simulink model "Spange_Thrust_simulation_4mode"  (R2016a)
settings: Solver=ode3  StartTime=0.0  StopTime=4  RelTol=1e-3
values from neighbouring files (symbols this model uses):
  C = [C1;C2;C3]    [Spange_init.m]
  D = 3.0/100    (= 0.03)    [Spange_init.m]
  eps_c = 5    [Spange_init.m]
  epsilon = 0.5    [Spange_init.m]
  hd = c2d(H1,0.1,'foh')    [Spange_init.m]
  hd2 = c2d(H2,0.01,'zoh')    [Spange_init.m]
  I_s = 0.05    [Spange_init.m]
  k_cc = 1    [Spange_init.m]
  K_omega = 0.3    [Spange_init.m]
  K_q1f = 0.0113    [Spange_init.m]
  K_q1r = K_q1f    (= 0.0113)    [Spange_init.m]
  K_q2f = 0.0117    [Spange_init.m]
  K_q2r = K_q2f    (= 0.0117)    [Spange_init.m]
  K_q3f = 0.0113    [Spange_init.m]
  K_q3r = K_q3f    (= 0.0113)    [Spange_init.m]
  K_T1f = 0.3763    [Spange_init.m]
  K_T1r = K_T1f    (= 0.3763)    [Spange_init.m]
  K_T2f = 0.3901    [Spange_init.m]
  K_T2r = K_T2f    (= 0.3901)    [Spange_init.m]
  K_T3f = 0.3776    [Spange_init.m]
  K_T3r = K_T3f    (= 0.3776)    [Spange_init.m]
  Kp = 0.3    [Spange_init.m]
  Max_Acceleration = 2    [Spange_init.m]
  Max_rotation = 12*sqrt(lambda)    [Spange_init.m]
  Max_thrust = 1.5034    [Spange_init.m]
  Min_thrust = -0.85    [Spange_init.m]
  mode = 4    [Spange_init.m]
  n_c = 5    [Spange_init.m]
  n_max = 64.6    [Spange_init.m]
  p_cc = 0.5    [Spange_init.m]
  Q_f0 = 0.3    [Spange_init.m]
  r_cc = 4    [Spange_init.m]
  Rho = Rho_m    (= 1000)    [Spange_init.m]
  td = [1;0;0]    [Spange_init.m]
  Thruster_control = 1    [Spange_init.m]
  ThrusterPosX = [Thruster.T1(1) Thruster.T2(1) Thruster.T3(1)]    [Spange_init.m]
  ThrusterPosY = [Thruster.T1(2) Thruster.T2(2) Thruster.T3(2)]    [Spange_init.m]
  u_e = [1 0 1 0 0 ... (first row only)    [Spange_init.m]
undefined symbols (not defined in the file or in its folder): Thruster
libraries: simulink_extras x16, simulink x8
(part 1 of 3)
settings Model: Creator=Joachim  LastModifiedBy=Joachim
settings DataIOCC: LimitDataPoints=on

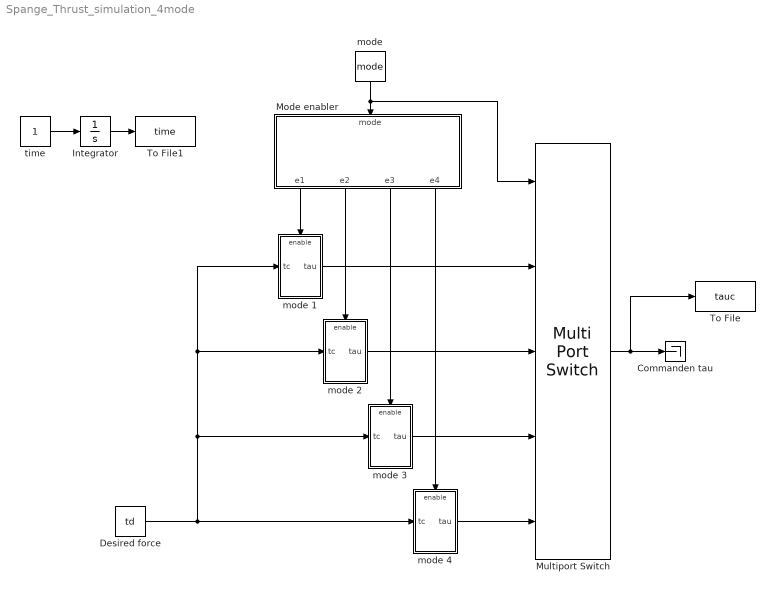
== system Spange_Thrust_simulation_4mode ==
  Commanden tau : Terminator
  Desired force : Constant  Value=td
  Integrator : Integrator
  Mode enabler : MATLAB Function  TreatAsAtomicUnit=on
  Multiport Switch : MultiPortSwitch  Inputs=4
  To File : ToFile  Filename=tauc  SaveFormat=Timeseries
  To File1 : ToFile  Filename=time  SaveFormat=Timeseries
  mode : Constant  Value=mode
  mode 1 : Subsystem
  mode 2 : Subsystem
  mode 3 : Subsystem
  mode 4 : Subsystem
  time : Constant
  wires:
  Mode enabler/4(e4) -> mode 4/Enable
  Desired force/1 -> mode 4/1(tc), mode 1/1(tc), mode 2/1(tc), mode 3/1(tc)
  Multiport Switch/1 -> To File/1, Commanden tau/1
  Mode enabler/1(e1) -> mode 1/Enable
  Mode enabler/2(e2) -> mode 2/Enable
  Mode enabler/3(e3) -> mode 3/Enable
  mode/1 -> Mode enabler/1(mode), Multiport Switch/1
  mode 3/1(tau) -> Multiport Switch/4
  mode 4/1(tau) -> Multiport Switch/5
  mode 2/1(tau) -> Multiport Switch/3
  mode 1/1(tau) -> Multiport Switch/2
  time/1 -> Integrator/1
  Integrator/1 -> To File1/1

== system Spange_Thrust_simulation_4mode/mode 1 ==
  note: Thust configuration 1
  tc : Inport
  Enable : EnablePort
  Ang com : Scope
  R2D : simulink_extras/Transformations/Radians to Degrees
  T(F,alpha) : Subsystem
  Thrus & angle aloc : Subsystem
  Thruster control : Subsystem
  To File : ToFile  Filename=Angm1  SaveFormat=Timeseries
  To File1 : ToFile  Filename=fm1  SaveFormat=Timeseries
  tau_Comm : Scope
  u_comm : Scope
  tau : Outport
  wires:
  Thrus & angle aloc/1(Td & angles) -> Thruster control/1("Desired thrust and angle ")
  tc/1 -> Thrus & angle aloc/2(tau)
  T(F,alpha)/1(Commanded tau) -> tau/1, tau_Comm/1
  R2D/1 -> Ang com/1
  Thruster control/2("Commanded thrust ") -> To File1/1, u_comm/1, Thrus & angle aloc/3(Thrust), T(F,alpha)/2(Commanded thrust)
  Thruster control/1(Commanded angle) -> T(F,alpha)/1(Commanded angle), To File/1, R2D/1, Thrus & angle aloc/1(Angles)

== system Spange_Thrust_simulation_4mode/mode 2 ==
  note: Thust configuration 2
  tc : Inport
  Enable : EnablePort
  Ang com : Scope
  R2D : simulink_extras/Transformations/Radians to Degrees
  T(F,alpha) : Subsystem
  Thrus & angle aloc : Subsystem
  Thruster control : Subsystem
  To File : ToFile  Filename=Angm2  SaveFormat=Timeseries
  To File1 : ToFile  Filename=fm2  SaveFormat=Timeseries
  tau_Comm : Scope
  u_comm : Scope
  tau : Outport
  wires:
  Thrus & angle aloc/1(Td & angles) -> Thruster control/1("Desired thrust and angle ")
  tc/1 -> Thrus & angle aloc/2(tau)
  T(F,alpha)/1(Commanded tau) -> tau/1, tau_Comm/1
  R2D/1 -> Ang com/1
  Thruster control/2("Commanded thrust ") -> To File1/1, u_comm/1, Thrus & angle aloc/3(Thrust), T(F,alpha)/2(Commanded thrust)
  Thruster control/1(Commanded angle) -> T(F,alpha)/1(Commanded angle), Thrus & angle aloc/1(Angles), To File/1, R2D/1

== system Spange_Thrust_simulation_4mode/mode 3 ==
  note: Thust configuration 3
  tc : Inport
  Enable : EnablePort
  Ang com : Scope
  R2D : simulink_extras/Transformations/Radians to Degrees
  T(F,alpha) : Subsystem
  Thrus & angle aloc : Subsystem
  Thruster control : Subsystem
  To File : ToFile  Filename=Angm3  SaveFormat=Timeseries
  To File1 : ToFile  Filename=fm3  SaveFormat=Timeseries
  tau_Comm : Scope
  u_comm : Scope
  tau : Outport
  wires:
  Thrus & angle aloc/1(Td & angles) -> Thruster control/1("Desired thrust and angle ")
  tc/1 -> Thrus & angle aloc/2(tau)
  T(F,alpha)/1(Commanded tau) -> tau/1, tau_Comm/1
  R2D/1 -> Ang com/1
  Thruster control/2("Commanded thrust ") -> To File1/1, u_comm/1, Thrus & angle aloc/3(Thrust), T(F,alpha)/2(Commanded thrust)
  Thruster control/1(Commanded angle) -> T(F,alpha)/1(Commanded angle), Thrus & angle aloc/1(Angles), To File/1, R2D/1

== system Spange_Thrust_simulation_4mode/mode 4 ==
  note: Thust configuration 4
  tc : Inport
  Enable : EnablePort
  Angles : Scope
  R2D : simulink_extras/Transformations/Radians to Degrees
  T(F,alpha) : Subsystem
  Tau comm : Scope
  Thrus & angle aloc : Subsystem
  Thruster control : Subsystem
  Thrusters : Scope
  To File : ToFile  Filename=Angm4  SaveFormat=Timeseries
  To File1 : ToFile  Filename=fm4  SaveFormat=Timeseries
  tau : Outport
  wires:
  Thrus & angle aloc/1(Td & angles) -> Thruster control/1("Desired thrust and angle ")
  tc/1 -> Thrus & angle aloc/2(tau)
  T(F,alpha)/1(Commanded tau) -> Tau comm/1, tau/1
  R2D/1 -> Angles/1
  Thruster control/2("Commanded thrust ") -> To File1/1, Thrusters/1, Thrus & angle aloc/3(Thrust), T(F,alpha)/2(Commanded thrust)
  Thruster control/1(Commanded angle) -> T(F,alpha)/1(Commanded angle), To File/1, R2D/1, Thrus & angle aloc/1(Angles)

== system Spange_Thrust_simulation_4mode/mode 1/T(F,alpha) ==
  Commanded angle : Inport
  Commanded thrust : Inport  Port=2
  MATLAB Function : MATLAB Function  TreatAsAtomicUnit=on
  Radians to Degrees : simulink_extras/Transformations/Radians to Degrees
  X-position Thruster : Constant  Value=[Thruster.T1(1)]
  Y-position Thruster : Constant  Value=[0]
  Commanded tau : Outport
  wires:
  Commanded angle/1 -> Radians to Degrees/1
  X-position Thruster/1 -> MATLAB Function/3(PosX)
  Y-position Thruster/1 -> MATLAB Function/4(PosY)
  MATLAB Function/1(actual_tau) -> Commanded tau/1
  Commanded thrust/1 -> MATLAB Function/1(thrust_actual)
  Radians to Degrees/1 -> MATLAB Function/2(alpha_actual)

== system Spange_Thrust_simulation_4mode/mode 1/Thrus & angle aloc ==
  Angles : Inport
  tau : Inport  Port=2
  Thrust : Inport  Port=3
  Delay : Delay  DelayLength=1  InitialCondition=[Thruster.T1(3)]
  Delay1 : Delay  DelayLength=1  InitialCondition=[0]
  Demux : Demux  Outputs=2
  For Each Subsystem : Subsystem  TreatAsAtomicUnit=on
  Mux : Mux  Inputs=3
  Mux2 : Mux  Inputs=2
  Radians to Degrees : simulink_extras/Transformations/Radians to Degrees
  Thrust and angle specified1 : Selector  InputPortWidth=2  IndexOptions=Index vector (dialog)  Indices=[2 1]  OutputSizes=1
  ThrustAllocation_Quadratic : S-Function  RequirementInfo={} %GIDa_a8b5f841_7abd_40df_aa52_0b8dc053099c  FunctionName=Spange_thrustallocationQuadratic_mode1  Parameters=u_e,Thruster,C  SFunctionDeploymentMode=off  EnableBusSupport=off
  constant angles : Constant  Value=[Thruster.T1(3)]
  Td & angles : Outport
  wires:
  tau/1 -> Mux/1
  Angles/1 -> Radians to Degrees/1
  Radians to Degrees/1 -> Delay/1
  Thrust/1 -> Delay1/1
  Delay/1 -> Mux/2
  Thrust and angle specified1/1 -> Td & angles/1
  Mux2/1 -> Thrust and angle specified1/1
  Demux/1 -> For Each Subsystem/1(Desired Angle)
  For Each Subsystem/1("Commanded angles [Rad] ") -> Mux2/1
  constant angles/1 -> For Each Subsystem/2("initial angle ")
  Demux/2 -> Mux2/2
  Delay1/1 -> Mux/3
  Mux/1 -> ThrustAllocation_Quadratic/1
  ThrustAllocation_Quadratic/1 -> Demux/1

== system Spange_Thrust_simulation_4mode/mode 1/Thruster control ==
  "Desired thrust and angle " : Inport
  Demux : Demux  Outputs=2
  Subsystem : Subsystem
  Thruster 1 : Subsystem
      settings: AttributesFormatString=%<MinAlgLoopOccurrences>
  Commanded angle : Outport
  "Commanded thrust " : Outport  Port=2
  wires:
  Demux/1 -> Thruster 1/1(Desired thrust 1)
  Thruster 1/1(Commanded thrust 1) -> Subsystem/1(Calculated thrust)
  Subsystem/1(Thrust from model) -> "Commanded thrust "/1
  Thruster 1/2(Commanded angle) -> Commanded angle/1
  Demux/2 -> Thruster 1/2(Desired Angle)
  "Desired thrust and angle "/1 -> Demux/1

== system Spange_Thrust_simulation_4mode/mode 2/T(F,alpha) ==
  Commanded angle : Inport
  Commanded thrust : Inport  Port=2
  MATLAB Function : MATLAB Function  TreatAsAtomicUnit=on
  Radians to Degrees : simulink_extras/Transformations/Radians to Degrees
  X-position Thruster : Constant  Value=[Thruster.T1(1) Thruster.T3(1)]
  Y-position Thruster : Constant  Value=[0 Thruster.T3(2)]
  Commanded tau : Outport
  wires:
  Commanded angle/1 -> Radians to Degrees/1
  X-position Thruster/1 -> MATLAB Function/3(PosX)
  Y-position Thruster/1 -> MATLAB Function/4(PosY)
  MATLAB Function/1(actual_tau) -> Commanded tau/1
  Commanded thrust/1 -> MATLAB Function/1(thrust_actual)
  Radians to Degrees/1 -> MATLAB Function/2(alpha_actual)

== system Spange_Thrust_simulation_4mode/mode 2/Thrus & angle aloc ==
  Angles : Inport
  tau : Inport  Port=2
  Thrust : Inport  Port=3
  "  Thrust calculated" : Selector  InputPortWidth=4  IndexOptions=Index vector (dialog)  Indices=[3 4]  OutputSizes=1
  " Angle calculated" : Selector  InputPortWidth=4  IndexOptions=Index vector (dialog)  Indices=[1 2]  OutputSizes=1
  Delay : Delay  DelayLength=1  InitialCondition=[Thruster.T1(3) Thruster.T3(3)]
  Delay1 : Delay  DelayLength=1  InitialCondition=[0,0]
  For Each Subsystem : Subsystem  TreatAsAtomicUnit=on
  Mux : Mux  Inputs=3
  Mux2 : Mux  Inputs=2
  Radians to Degrees : simulink_extras/Transformations/Radians to Degrees
  Thrust and angle specified1 : Selector  InputPortWidth=4  IndexOptions=Index vector (dialog)  Indices=[3 1 4 2]  OutputSizes=1
  ThrustAllocation_Quadratic : S-Function  RequirementInfo={} %GIDa_7aa52336_02c6_4a01_b2d7_61ed65dc0b87  FunctionName=Spange_thrustallocationQuadratic_mode2  Parameters=u_e,Thruster,C  SFunctionDeploymentMode=off  EnableBusSupport=off
  constant angles : Constant  Value=[Thruster.T1(3) Thruster.T3(3)]
  Td & angles : Outport
  wires:
  tau/1 -> Mux/1
  Angles/1 -> Radians to Degrees/1
  Radians to Degrees/1 -> Delay/1
  Thrust/1 -> Delay1/1
  Delay/1 -> Mux/2
  Thrust and angle specified1/1 -> Td & angles/1
  Mux2/1 -> Thrust and angle specified1/1
  " Angle calculated"/1 -> For Each Subsystem/1(Desired Angle)
  For Each Subsystem/1("Commanded angles [Rad] ") -> Mux2/1
  constant angles/1 -> For Each Subsystem/2("initial angle ")
  "  Thrust calculated"/1 -> Mux2/2
  ThrustAllocation_Quadratic/1 -> " Angle calculated"/1, "  Thrust calculated"/1
  Delay1/1 -> Mux/3
  Mux/1 -> ThrustAllocation_Quadratic/1

== system Spange_Thrust_simulation_4mode/mode 2/Thruster control ==
  "Desired thrust and angle " : Inport
  Demux : Demux
  Mux : Mux
  Selecting Actual thrust : Selector  InputPortWidth=4  IndexOptions=Index vector (dialog)  Indices=[1 3]  OutputSizes=1
  Selecting actual angle : Selector  InputPortWidth=4  IndexOptions=Index vector (dialog)  Indices=[2 4]  OutputSizes=1
  Subsystem : Subsystem
  Thruster 1 : Subsystem
      settings: AttributesFormatString=%<MinAlgLoopOccurrences>
  Thruster 3 : Subsystem
      settings: AttributesFormatString=%<MinAlgLoopOccurrences>
  Commanded angle : Outport
  "Commanded thrust " : Outport  Port=2
  wires:
  Demux/1 -> Thruster 1/1(Desired thrust 1)
  Selecting Actual thrust/1 -> Subsystem/1(Calculated thrust)
  Subsystem/1(Thrust from model) -> "Commanded thrust "/1
  Selecting actual angle/1 -> Commanded angle/1
  Thruster 1/2(Commanded angle) -> Mux/2
  Demux/2 -> Thruster 1/2(Desired Angle)
  Mux/1 -> Selecting Actual thrust/1, Selecting actual angle/1
  Thruster 3/2(Commanded angle) -> Mux/4
  Thruster 3/1("Commanded thrust ") -> Mux/3
  Thruster 1/1(Commanded thrust 1) -> Mux/1
  Demux/4 -> Thruster 3/2(Desired Angle)
  Demux/3 -> Thruster 3/1(Desired thrust 1)
  "Desired thrust and angle "/1 -> Demux/1

== system Spange_Thrust_simulation_4mode/mode 3/T(F,alpha) ==
  Commanded angle : Inport
  Commanded thrust : Inport  Port=2
  MATLAB Function : MATLAB Function  TreatAsAtomicUnit=on
  Radians to Degrees : simulink_extras/Transformations/Radians to Degrees
  X-position Thruster : Constant  Value=[Thruster.T1(1) Thruster.T2(1)]
  Y-position Thruster : Constant  Value=[Thruster.T1(2) Thruster.T2(2)]
  Commanded tau : Outport
  wires:
  Commanded angle/1 -> Radians to Degrees/1
  X-position Thruster/1 -> MATLAB Function/3(PosX)
  Y-position Thruster/1 -> MATLAB Function/4(PosY)
  MATLAB Function/1(actual_tau) -> Commanded tau/1
  Commanded thrust/1 -> MATLAB Function/1(thrust_actual)
  Radians to Degrees/1 -> MATLAB Function/2(alpha_actual)

== system Spange_Thrust_simulation_4mode/mode 3/Thrus & angle aloc ==
  Angles : Inport
  tau : Inport  Port=2
  Thrust : Inport  Port=3
  "  Thrust calculated" : Selector  InputPortWidth=4  IndexOptions=Index vector (dialog)  Indices=[3 4]  OutputSizes=1
  " Angle calculated" : Selector  InputPortWidth=4  IndexOptions=Index vector (dialog)  Indices=[1 2]  OutputSizes=1
  Delay : Delay  DelayLength=1  InitialCondition=[Thruster.T1(3) Thruster.T2(3)]
  Delay1 : Delay  DelayLength=1  InitialCondition=[0,0]
  For Each Subsystem : Subsystem  TreatAsAtomicUnit=on
  Mux : Mux  Inputs=3
  Mux2 : Mux  Inputs=2
  Radians to Degrees : simulink_extras/Transformations/Radians to Degrees
  Thrust and angle specified1 : Selector  InputPortWidth=4  IndexOptions=Index vector (dialog)  Indices=[3 1 4 2]  OutputSizes=1
  ThrustAllocation_Quadratic : S-Function  RequirementInfo={} %GIDa_a7b51f9f_920d_4275_ac87_dfaea04df3fe  FunctionName=Spange_thrustallocationQuadratic_mode3  Parameters=u_e,Thruster,C  SFunctionDeploymentMode=off  EnableBusSupport=off
  constant angles : Constant  Value=[Thruster.T1(3) Thruster.T2(3)]
  Td & angles : Outport
  wires:
  tau/1 -> Mux/1
  Angles/1 -> Radians to Degrees/1
  Radians to Degrees/1 -> Delay/1
  Thrust/1 -> Delay1/1
  Delay/1 -> Mux/2
  Thrust and angle specified1/1 -> Td & angles/1
  Mux2/1 -> Thrust and angle specified1/1
  " Angle calculated"/1 -> For Each Subsystem/1(Desired Angle)
  For Each Subsystem/1("Commanded angles [Rad] ") -> Mux2/1
  constant angles/1 -> For Each Subsystem/2("initial angle ")
  "  Thrust calculated"/1 -> Mux2/2
  ThrustAllocation_Quadratic/1 -> " Angle calculated"/1, "  Thrust calculated"/1
  Delay1/1 -> Mux/3
  Mux/1 -> ThrustAllocation_Quadratic/1

== system Spange_Thrust_simulation_4mode/mode 3/Thruster control ==
  "Desired thrust and angle " : Inport
  Demux : Demux
  Mux : Mux
  Selecting Actual thrust : Selector  InputPortWidth=4  IndexOptions=Index vector (dialog)  Indices=[1 3]  OutputSizes=1
  Selecting actual angle : Selector  InputPortWidth=4  IndexOptions=Index vector (dialog)  Indices=[2 4]  OutputSizes=1
  Subsystem : Subsystem
  Thruster 1 : Subsystem
      settings: AttributesFormatString=%<MinAlgLoopOccurrences>
  Thruster 2 : Subsystem
      settings: AttributesFormatString=%<MinAlgLoopOccurrences>
  Commanded angle : Outport
  "Commanded thrust " : Outport  Port=2
  wires:
  Demux/1 -> Thruster 1/1(Desired thrust 1)
  Selecting Actual thrust/1 -> Subsystem/1(Calculated thrust)
  Subsystem/1(Thrust from model) -> "Commanded thrust "/1
  Selecting actual angle/1 -> Commanded angle/1
  Thruster 1/2(Commanded angle) -> Mux/2
  Demux/2 -> Thruster 1/2(Desired Angle)
  Mux/1 -> Selecting Actual thrust/1, Selecting actual angle/1
  Thruster 2/2(Commanded angle) -> Mux/4
  Thruster 2/1(Commanded thrust 1) -> Mux/3
  Thruster 1/1(Commanded thrust 1) -> Mux/1
  Demux/4 -> Thruster 2/2(Desired Angle)
  Demux/3 -> Thruster 2/1(Desired thrust 1)
  "Desired thrust and angle "/1 -> Demux/1

== system Spange_Thrust_simulation_4mode/mode 4/T(F,alpha) ==
  Commanded angle : Inport
  Commanded thrust : Inport  Port=2
  MATLAB Function : MATLAB Function  TreatAsAtomicUnit=on
  Radians to Degrees : simulink_extras/Transformations/Radians to Degrees
  Commanded tau : Outport
  wires:
  Commanded angle/1 -> Radians to Degrees/1
  MATLAB Function/1(actual_tau) -> Commanded tau/1
  Commanded thrust/1 -> MATLAB Function/1(thrust_actual)
  Radians to Degrees/1 -> MATLAB Function/2(alpha_actual)

== system Spange_Thrust_simulation_4mode/mode 4/Thrus & angle aloc ==
  Angles : Inport
  tau : Inport  Port=2
  Thrust : Inport  Port=3
  "  Thrust calculated" : Selector  InputPortWidth=6  IndexOptions=Index vector (dialog)  Indices=[4 5 6]  OutputSizes=1
  " Angle calculated" : Selector  InputPortWidth=6  IndexOptions=Index vector (dialog)  Indices=[1 2 3]  OutputSizes=1
  Delay : Delay  DelayLength=1  InitialCondition=[Thruster.T1(3) Thruster.T2(3) Thruster.T3(3)]
  Delay1 : Delay  DelayLength=1  InitialCondition=[0,0,0]
  For Each Subsystem : Subsystem  TreatAsAtomicUnit=on
  Mux : Mux  Inputs=3
  Mux2 : Mux  Inputs=2
  Radians to Degrees : simulink_extras/Transformations/Radians to Degrees
  Thrust and angle specified1 : Selector  InputPortWidth=6  IndexOptions=Index vector (dialog)  Indices=[4 1 5 2 6 3]  OutputSizes=1
  ThrustAllocation_Quadratic : S-Function  RequirementInfo={} %GIDa_b9c7dd03_57d1_40a3_b341_131bae047cf5  FunctionName=Spange_thrustallocationQuadratic_mode4  Parameters=u_e,Thruster,C  SFunctionDeploymentMode=off  EnableBusSupport=off
  constant angles : Constant  Value=[Thruster.T1(3) Thruster.T2(3) Thruster.T3(3)]
  pseudoinverse : MATLAB Function  Commented=on  TreatAsAtomicUnit=on
  Td & angles : Outport
  wires:
  tau/1 -> Mux/1
  Angles/1 -> Radians to Degrees/1
  Radians to Degrees/1 -> Delay/1
  Thrust/1 -> Delay1/1
  Delay/1 -> Mux/2
  Thrust and angle specified1/1 -> Td & angles/1
  Mux2/1 -> Thrust and angle specified1/1
  " Angle calculated"/1 -> For Each Subsystem/1(Desired Angle)
  For Each Subsystem/1("Commanded angles [Rad] ") -> Mux2/1
  constant angles/1 -> For Each Subsystem/2("initial angle ")
  "  Thrust calculated"/1 -> Mux2/2
  ThrustAllocation_Quadratic/1 -> "  Thrust calculated"/1, " Angle calculated"/1
  Delay1/1 -> Mux/3
  Mux/1 -> ThrustAllocation_Quadratic/1

== system Spange_Thrust_simulation_4mode/mode 4/Thruster control ==
  "Desired thrust and angle " : Inport
  Demux : Demux  Outputs=6
  Mux : Mux  Inputs=6
  Selecting Actual thrust : Selector  InputPortWidth=6  IndexOptions=Index vector (dialog)  Indices=[1 3 5]  OutputSizes=1
  Selecting actual angle : Selector  InputPortWidth=6  IndexOptions=Index vector (dialog)  Indices=[2 4 6]  OutputSizes=1
  Subsystem : Subsystem
  Thruster 1 : Subsystem
      settings: AttributesFormatString=%<MinAlgLoopOccurrences>
  Thruster 2 : Subsystem
      settings: AttributesFormatString=%<MinAlgLoopOccurrences>
  Thruster 3 : Subsystem
      settings: AttributesFormatString=%<MinAlgLoopOccurrences>
  Commanded angle : Outport
  "Commanded thrust " : Outport  Port=2
  wires:
  Demux/1 -> Thruster 1/1(Desired thrust 1)
  Selecting Actual thrust/1 -> Subsystem/1(Calculated thrust)
  Subsystem/1(Thrust from model) -> "Commanded thrust "/1
  Selecting actual angle/1 -> Commanded angle/1
  Thruster 1/2(Commanded angle) -> Mux/2
  Demux/2 -> Thruster 1/2(Desired Angle)
  Mux/1 -> Selecting Actual thrust/1, Selecting actual angle/1
  Thruster 3/2(Commanded angle) -> Mux/6
  Thruster 3/1("Commanded thrust ") -> Mux/5
  Thruster 2/2(Commanded angle) -> Mux/4
  Thruster 2/1(Commanded thrust 1) -> Mux/3
  Thruster 1/1(Commanded thrust 1) -> Mux/1
  Demux/6 -> Thruster 3/2(Desired Angle)
  Demux/5 -> Thruster 3/1(Desired thrust 1)
  Demux/4 -> Thruster 2/2(Desired Angle)
  Demux/3 -> Thruster 2/1(Desired thrust 1)
  "Desired thrust and angle "/1 -> Demux/1

== system Spange_Thrust_simulation_4mode/mode 1/Thrus & angle aloc/For Each Subsystem ==
  Desired Angle : Inport
  "initial angle " : Inport  Port=2
  Degrees to Radians : simulink_extras/Transformations/Degrees to Radians
  Ensures fastest way is chosen : MATLAB Function  TreatAsAtomicUnit=on
  Integrator : Integrator  ExternalReset=either  InitialConditionSource=external
  MATLAB Function : MATLAB Function  TreatAsAtomicUnit=on
  Max Rotation Rate : Saturate  UpperLimit=Max_rotation  LowerLimit=-Max_rotation
  constant : Constant  Value=0
  "Commanded angles [Rad] " : Outport
  wires:
  Degrees to Radians/1 -> MATLAB Function/1(angle)
  MATLAB Function/1(y) -> "Commanded angles [Rad] "/1
  Integrator/1 -> Degrees to Radians/1, Ensures fastest way is chosen/2(actual)  "angle"
  "initial angle "/1 -> Integrator/3
  Max Rotation Rate/1 -> Integrator/1
  Ensures fastest way is chosen/1(psi_D) -> Max Rotation Rate/1
  Desired Angle/1 -> Ensures fastest way is chosen/1(desired)
  constant/1 -> Integrator/2

== system Spange_Thrust_simulation_4mode/mode 1/Thruster control/Subsystem ==
  Calculated thrust : Inport
  Saturation 1 : Saturate  UpperLimit=Max_thrust  LowerLimit=Min_thrust
  Thrust from model : Outport
  wires:
  Saturation 1/1 -> Thrust from model/1
  Calculated thrust/1 -> Saturation 1/1

== system Spange_Thrust_simulation_4mode/mode 1/Thruster control/Thruster 1 ==
  Desired thrust 1 : Inport
  Desired Angle : Inport  Port=2
  Constant : Constant  Value=hd2.den{1,1}
  Constant1 : Constant  Value=hd2.num{1,1}
  Discrete Transfer Fcn : DiscreteTransferFcn  NumeratorSource=Input port  DenominatorSource=Input port  Denominator=[0.2 1]  SampleTime=0.01  a0EqualsOne=on
      settings: InputPortMap=u0,p1,p3
  Losses (placeholder) : Constant  Value=0
  Propeller Hydrodynamics : Subsystem
  Shaft dynamics : Subsystem
  Thruster control : Subsystem
  Commanded thrust 1 : Outport
  Commanded angle : Outport  Port=2
  wires:
  Desired thrust 1/1 -> Thruster control/1("T_d ")
  Discrete Transfer Fcn/1 -> Shaft dynamics/1(Qm)
  Propeller Hydrodynamics/2(Qa) -> Shaft dynamics/2(Qa)
  Shaft dynamics/1(n) -> Propeller Hydrodynamics/2(n), Thruster control/2(n)
  Constant/1 -> Discrete Transfer Fcn/3
  Constant1/1 -> Discrete Transfer Fcn/2
  Desired Angle/1 -> Commanded angle/1
  Thruster control/1(Qc) -> Discrete Transfer Fcn/1
  Propeller Hydrodynamics/1(Ta) -> Commanded thrust 1/1
  Losses (placeholder)/1 -> Propeller Hydrodynamics/1(env)

== system Spange_Thrust_simulation_4mode/mode 2/Thrus & angle aloc/For Each Subsystem ==
  Desired Angle : Inport  Partition=on  PartitionDimension=1  PartitionWidth=1
  "initial angle " : Inport  Port=2  Partition=on  PartitionDimension=1  PartitionWidth=1
  Degrees to Radians : simulink_extras/Transformations/Degrees to Radians
  Ensures fastest way is chosen : MATLAB Function  TreatAsAtomicUnit=on
  For Each : ForEach  DisableCoverage=on  IndexMode=One-based
  Integrator : Integrator  ExternalReset=either  InitialConditionSource=external
  MATLAB Function : MATLAB Function  TreatAsAtomicUnit=on
  Max Rotation Rate : Saturate  UpperLimit=Max_rotation  LowerLimit=-Max_rotation
  constant : Constant  Value=0
  "Commanded angles [Rad] " : Outport  ConcatenationDimension=1
  wires:
  Degrees to Radians/1 -> MATLAB Function/1(angle)
  MATLAB Function/1(y) -> "Commanded angles [Rad] "/1
  Integrator/1 -> Degrees to Radians/1, Ensures fastest way is chosen/2(actual)  "angle"
  "initial angle "/1 -> Integrator/3
  Max Rotation Rate/1 -> Integrator/1
  Ensures fastest way is chosen/1(psi_D) -> Max Rotation Rate/1
  Desired Angle/1 -> Ensures fastest way is chosen/1(desired)
  constant/1 -> Integrator/2

== system Spange_Thrust_simulation_4mode/mode 2/Thruster control/Subsystem ==
  Calculated thrust : Inport
  Demux : Demux  Outputs=2
  Mux : Mux  Inputs=2
  Saturation 1 : Saturate  UpperLimit=Max_thrust  LowerLimit=Min_thrust
  Saturation 2 : Saturate  UpperLimit=Max_thrust  LowerLimit=Min_thrust
  Thrust from model : Outport
  wires:
  Saturation 2/1 -> Mux/2
  Saturation 1/1 -> Mux/1
  Mux/1 -> Thrust from model/1
  Demux/2 -> Saturation 2/1
  Demux/1 -> Saturation 1/1
  Calculated thrust/1 -> Demux/1

== system Spange_Thrust_simulation_4mode/mode 2/Thruster control/Thruster 1 ==
  Desired thrust 1 : Inport
  Desired Angle : Inport  Port=2
  Constant : Constant  Value=hd2.den{1,1}
  Constant1 : Constant  Value=hd2.num{1,1}
  Discrete Transfer Fcn : DiscreteTransferFcn  NumeratorSource=Input port  DenominatorSource=Input port  Denominator=[0.2 1]  SampleTime=0.01  a0EqualsOne=on
      settings: InputPortMap=u0,p1,p3
  Losses (placeholder) : Constant  Value=0
  Propeller Hydrodynamics : Subsystem
  Shaft dynamics : Subsystem
  Thruster control : Subsystem
  Commanded thrust 1 : Outport
  Commanded angle : Outport  Port=2
  wires:
  Desired thrust 1/1 -> Thruster control/1("T_d ")
  Discrete Transfer Fcn/1 -> Shaft dynamics/1(Qm)
  Propeller Hydrodynamics/2(Qa) -> Shaft dynamics/2(Qa)
  Shaft dynamics/1(n) -> Propeller Hydrodynamics/2(n), Thruster control/2(n)
  Constant/1 -> Discrete Transfer Fcn/3
  Constant1/1 -> Discrete Transfer Fcn/2
  Desired Angle/1 -> Commanded angle/1
  Thruster control/1(Qc) -> Discrete Transfer Fcn/1
  Propeller Hydrodynamics/1(Ta) -> Commanded thrust 1/1
  Losses (placeholder)/1 -> Propeller Hydrodynamics/1(env)

== system Spange_Thrust_simulation_4mode/mode 2/Thruster control/Thruster 3 ==
  Desired thrust 1 : Inport
  Desired Angle : Inport  Port=2
  Constant : Constant  Value=hd2.den{1,1}
  Constant1 : Constant  Value=hd2.num{1,1}
  Discrete Transfer Fcn : DiscreteTransferFcn  NumeratorSource=Input port  DenominatorSource=Input port  Denominator=[0.2 1]  SampleTime=0.01  a0EqualsOne=on
      settings: InputPortMap=u0,p1,p3
  Losses (placeholder) : Constant  Value=0
  Propeller Hydrodynamics : Subsystem
  Shaft dynamics : Subsystem
  Thruster control : Subsystem
  "Commanded thrust " : Outport
  Commanded angle : Outport  Port=2
  wires:
  Propeller Hydrodynamics/2(Qa) -> Shaft dynamics/2(Qa)
  Shaft dynamics/1(n) -> Propeller Hydrodynamics/2(n), Thruster control/2(n)
  Constant/1 -> Discrete Transfer Fcn/3
  Constant1/1 -> Discrete Transfer Fcn/2
  Desired Angle/1 -> Commanded angle/1
  Propeller Hydrodynamics/1(Ta) -> "Commanded thrust "/1
  Desired thrust 1/1 -> Thruster control/1("T_d ")
  Discrete Transfer Fcn/1 -> Shaft dynamics/1(Qm)
  Thruster control/1(Qc) -> Discrete Transfer Fcn/1
  Losses (placeholder)/1 -> Propeller Hydrodynamics/1(env)

== system Spange_Thrust_simulation_4mode/mode 3/Thrus & angle aloc/For Each Subsystem ==
  Desired Angle : Inport  Partition=on  PartitionDimension=1  PartitionWidth=1
  "initial angle " : Inport  Port=2  Partition=on  PartitionDimension=1  PartitionWidth=1
  Degrees to Radians : simulink_extras/Transformations/Degrees to Radians
  Ensures fastest way is chosen : MATLAB Function  TreatAsAtomicUnit=on
  For Each : ForEach  DisableCoverage=on  IndexMode=One-based
  Integrator : Integrator  ExternalReset=either  InitialConditionSource=external
  MATLAB Function : MATLAB Function  TreatAsAtomicUnit=on
  Max Rotation Rate : Saturate  UpperLimit=Max_rotation  LowerLimit=-Max_rotation
  constant : Constant  Value=0
  "Commanded angles [Rad] " : Outport  ConcatenationDimension=1
  wires:
  Degrees to Radians/1 -> MATLAB Function/1(angle)
  MATLAB Function/1(y) -> "Commanded angles [Rad] "/1
  Integrator/1 -> Degrees to Radians/1, Ensures fastest way is chosen/2(actual)  "angle"
  "initial angle "/1 -> Integrator/3
  Max Rotation Rate/1 -> Integrator/1
  Ensures fastest way is chosen/1(psi_D) -> Max Rotation Rate/1
  Desired Angle/1 -> Ensures fastest way is chosen/1(desired)
  constant/1 -> Integrator/2

== system Spange_Thrust_simulation_4mode/mode 3/Thruster control/Subsystem ==
  Calculated thrust : Inport
  Demux : Demux  Outputs=2
  Mux : Mux  Inputs=2
  Saturation 1 : Saturate  UpperLimit=Max_thrust  LowerLimit=Min_thrust
  Saturation 2 : Saturate  UpperLimit=Max_thrust  LowerLimit=Min_thrust
  Thrust from model : Outport
  wires:
  Saturation 2/1 -> Mux/2
  Saturation 1/1 -> Mux/1
  Mux/1 -> Thrust from model/1
  Demux/2 -> Saturation 2/1
  Demux/1 -> Saturation 1/1
  Calculated thrust/1 -> Demux/1

== system Spange_Thrust_simulation_4mode/mode 3/Thruster control/Thruster 1 ==
  Desired thrust 1 : Inport
  Desired Angle : Inport  Port=2
  Constant : Constant  Value=hd2.den{1,1}
  Constant1 : Constant  Value=hd2.num{1,1}
  Discrete Transfer Fcn : DiscreteTransferFcn  NumeratorSource=Input port  DenominatorSource=Input port  Denominator=[0.2 1]  SampleTime=0.01  a0EqualsOne=on
      settings: InputPortMap=u0,p1,p3
  Losses (placeholder) : Constant  Value=0
  Propeller Hydrodynamics : Subsystem
  Shaft dynamics : Subsystem
  Thruster control : Subsystem
  Commanded thrust 1 : Outport
  Commanded angle : Outport  Port=2
  wires:
  Desired thrust 1/1 -> Thruster control/1("T_d ")
  Discrete Transfer Fcn/1 -> Shaft dynamics/1(Qm)
  Propeller Hydrodynamics/2(Qa) -> Shaft dynamics/2(Qa)
  Shaft dynamics/1(n) -> Propeller Hydrodynamics/2(n), Thruster control/2(n)
  Constant/1 -> Discrete Transfer Fcn/3
  Constant1/1 -> Discrete Transfer Fcn/2
  Desired Angle/1 -> Commanded angle/1
  Thruster control/1(Qc) -> Discrete Transfer Fcn/1
  Propeller Hydrodynamics/1(Ta) -> Commanded thrust 1/1
  Losses (placeholder)/1 -> Propeller Hydrodynamics/1(env)

== system Spange_Thrust_simulation_4mode/mode 3/Thruster control/Thruster 2 ==
  Desired thrust 1 : Inport
  Desired Angle : Inport  Port=2
  Constant : Constant  Value=hd2.den{1,1}
  Constant1 : Constant  Value=hd2.num{1,1}
  Discrete Transfer Fcn : DiscreteTransferFcn  NumeratorSource=Input port  DenominatorSource=Input port  Denominator=[0.2 1]  SampleTime=0.01  a0EqualsOne=on
      settings: InputPortMap=u0,p1,p3
  Losses (placeholder) : Constant  Value=0
  Propeller Hydrodynamics : Subsystem
  Shaft dynamics : Subsystem
  Thruster control : Subsystem
  Commanded thrust 1 : Outport
  Commanded angle : Outport  Port=2
  wires:
  Propeller Hydrodynamics/2(Qa) -> Shaft dynamics/2(Qa)
  Shaft dynamics/1(n) -> Propeller Hydrodynamics/2(n), Thruster control/2(n)
  Constant/1 -> Discrete Transfer Fcn/3
  Constant1/1 -> Discrete Transfer Fcn/2
  Desired Angle/1 -> Commanded angle/1
  Propeller Hydrodynamics/1(Ta) -> Commanded thrust 1/1
  Desired thrust 1/1 -> Thruster control/1("T_d ")
  Discrete Transfer Fcn/1 -> Shaft dynamics/1(Qm)
  Thruster control/1(Qc) -> Discrete Transfer Fcn/1
  Losses (placeholder)/1 -> Propeller Hydrodynamics/1(env)

== system Spange_Thrust_simulation_4mode/mode 4/Thrus & angle aloc/For Each Subsystem ==
  Desired Angle : Inport  Partition=on  PartitionDimension=1  PartitionWidth=1
  "initial angle " : Inport  Port=2  Partition=on  PartitionDimension=1  PartitionWidth=1
  Degrees to Radians : simulink_extras/Transformations/Degrees to Radians
  Ensures fastest way is chosen : MATLAB Function  TreatAsAtomicUnit=on
  For Each : ForEach  DisableCoverage=on  IndexMode=One-based
  Integrator : Integrator  ExternalReset=either  InitialConditionSource=external
  MATLAB Function : MATLAB Function  TreatAsAtomicUnit=on
  Max Rotation Rate : Saturate  UpperLimit=Max_rotation  LowerLimit=-Max_rotation
  constant : Constant  Value=0
  "Commanded angles [Rad] " : Outport  ConcatenationDimension=1
  wires:
  Degrees to Radians/1 -> MATLAB Function/1(angle)
  MATLAB Function/1(y) -> "Commanded angles [Rad] "/1
  Integrator/1 -> Degrees to Radians/1, Ensures fastest way is chosen/2(actual)  "angle"
  "initial angle "/1 -> Integrator/3
  Max Rotation Rate/1 -> Integrator/1
  Ensures fastest way is chosen/1(psi_D) -> Max Rotation Rate/1
  Desired Angle/1 -> Ensures fastest way is chosen/1(desired)
  constant/1 -> Integrator/2

== system Spange_Thrust_simulation_4mode/mode 4/Thruster control/Subsystem ==
  Calculated thrust : Inport
  Demux : Demux  Outputs=3
  Mux : Mux  Inputs=3
  Saturation 1 : Saturate  UpperLimit=Max_thrust  LowerLimit=Min_thrust
  Saturation 2 : Saturate  UpperLimit=Max_thrust  LowerLimit=Min_thrust
  Saturation 3 : Saturate  UpperLimit=Max_thrust  LowerLimit=Min_thrust
  Thrust from model : Outport
  wires:
  Saturation 2/1 -> Mux/2
  Saturation 3/1 -> Mux/3
  Saturation 1/1 -> Mux/1
  Mux/1 -> Thrust from model/1
  Demux/3 -> Saturation 3/1
  Demux/2 -> Saturation 2/1
  Demux/1 -> Saturation 1/1
  Calculated thrust/1 -> Demux/1

== system Spange_Thrust_simulation_4mode/mode 4/Thruster control/Thruster 1 ==
  Desired thrust 1 : Inport
  Desired Angle : Inport  Port=2
  Constant : Constant  Value=hd2.den{1,1}
  Constant1 : Constant  Value=hd2.num{1,1}
  Discrete Transfer Fcn : DiscreteTransferFcn  NumeratorSource=Input port  DenominatorSource=Input port  Denominator=[0.2 1]  SampleTime=0.01  a0EqualsOne=on
      settings: InputPortMap=u0,p1,p3
  Losses (placeholder) : Constant  Value=0
  Propeller Hydrodynamics : Subsystem
  Shaft dynamics : Subsystem
  Thruster control : Subsystem
  Commanded thrust 1 : Outport
  Commanded angle : Outport  Port=2
  wires:
  Desired thrust 1/1 -> Thruster control/1("T_d ")
  Discrete Transfer Fcn/1 -> Shaft dynamics/1(Qm)
  Propeller Hydrodynamics/2(Qa) -> Shaft dynamics/2(Qa)
  Shaft dynamics/1(n) -> Propeller Hydrodynamics/2(n), Thruster control/2(n)
  Constant/1 -> Discrete Transfer Fcn/3
  Constant1/1 -> Discrete Transfer Fcn/2
  Desired Angle/1 -> Commanded angle/1
  Thruster control/1(Qc) -> Discrete Transfer Fcn/1
  Propeller Hydrodynamics/1(Ta) -> Commanded thrust 1/1
  Losses (placeholder)/1 -> Propeller Hydrodynamics/1(env)

== system Spange_Thrust_simulation_4mode/mode 4/Thruster control/Thruster 2 ==
  Desired thrust 1 : Inport
  Desired Angle : Inport  Port=2
  Constant : Constant  Value=hd2.den{1,1}
  Constant1 : Constant  Value=hd2.num{1,1}
  Discrete Transfer Fcn : DiscreteTransferFcn  NumeratorSource=Input port  DenominatorSource=Input port  Denominator=[0.2 1]  SampleTime=0.01  a0EqualsOne=on
      settings: InputPortMap=u0,p1,p3
  Losses (placeholder) : Constant  Value=0
  Propeller Hydrodynamics : Subsystem
  Shaft dynamics : Subsystem
  Thruster control : Subsystem
  Commanded thrust 1 : Outport
  Commanded angle : Outport  Port=2
  wires:
  Propeller Hydrodynamics/2(Qa) -> Shaft dynamics/2(Qa)
  Shaft dynamics/1(n) -> Propeller Hydrodynamics/2(n), Thruster control/2(n)
  Constant/1 -> Discrete Transfer Fcn/3
  Constant1/1 -> Discrete Transfer Fcn/2
  Desired Angle/1 -> Commanded angle/1
  Propeller Hydrodynamics/1(Ta) -> Commanded thrust 1/1
  Desired thrust 1/1 -> Thruster control/1("T_d ")
  Discrete Transfer Fcn/1 -> Shaft dynamics/1(Qm)
  Thruster control/1(Qc) -> Discrete Transfer Fcn/1
  Losses (placeholder)/1 -> Propeller Hydrodynamics/1(env)

== system Spange_Thrust_simulation_4mode/mode 4/Thruster control/Thruster 3 ==
  Desired thrust 1 : Inport
  Desired Angle : Inport  Port=2
  Constant : Constant  Value=hd2.den{1,1}
  Constant1 : Constant  Value=hd2.num{1,1}
  Discrete Transfer Fcn : DiscreteTransferFcn  NumeratorSource=Input port  DenominatorSource=Input port  Denominator=[0.2 1]  SampleTime=0.01  a0EqualsOne=on
      settings: InputPortMap=u0,p1,p3
  Losses (placeholder) : Constant  Value=0
  Propeller Hydrodynamics : Subsystem
  Shaft dynamics : Subsystem
  Thruster control : Subsystem
  "Commanded thrust " : Outport
  Commanded angle : Outport  Port=2
  wires:
  Propeller Hydrodynamics/2(Qa) -> Shaft dynamics/2(Qa)
  Shaft dynamics/1(n) -> Propeller Hydrodynamics/2(n), Thruster control/2(n)
  Constant/1 -> Discrete Transfer Fcn/3
  Constant1/1 -> Discrete Transfer Fcn/2
  Desired Angle/1 -> Commanded angle/1
  Propeller Hydrodynamics/1(Ta) -> "Commanded thrust "/1
  Desired thrust 1/1 -> Thruster control/1("T_d ")
  Discrete Transfer Fcn/1 -> Shaft dynamics/1(Qm)
  Thruster control/1(Qc) -> Discrete Transfer Fcn/1
  Losses (placeholder)/1 -> Propeller Hydrodynamics/1(env)

== system Spange_Thrust_simulation_4mode/mode 1/Thruster control/Thruster 1/Propeller Hydrodynamics ==
  env : Inport
  n : Inport  Port=2
  Actual Force and Torque : MATLAB Function  TreatAsAtomicUnit=on
  D1 : Constant  Value=D
  Kq1 : Constant  Value=K_q1f
  Kqr1 : Constant  Value=K_q1r
  Ktf : Constant  Value=K_T1f
  Ktr : Constant  Value=K_T1r
  Rho1 : Constant  Value=Rho
  eps_c1 : Constant  Value=eps_c
  Ta : Outport
  Qa : Outport  Port=2
  wires:
  eps_c1/1 -> Actual Force and Torque/8(eps_c)
  Kqr1/1 -> Actual Force and Torque/5(Kqr)
  Ktr/1 -> Actual Force and Torque/4(Ktr)
  Actual Force and Torque/1(Ta) -> Ta/1
  Ktf/1 -> Actual Force and Torque/3(Kt)
  env/1 -> Actual Force and Torque/9(env)
  Rho1/1 -> Actual Force and Torque/6(Rho)
  Actual Force and Torque/2(Qa) -> Qa/1
  Kq1/1 -> Actual Force and Torque/2(Kq)
  D1/1 -> Actual Force and Torque/7(D)
  n/1 -> Actual Force and Torque/1(n)

== system Spange_Thrust_simulation_4mode/mode 1/Thruster control/Thruster 1/Shaft dynamics ==
  Qm : Inport
  Qa : Inport  Port=2
  Constant : Constant  Value=0
  Finding rotation speed : Gain  Gain=1/(2*pi*I_s)
  Integrator : Integrator  ExternalReset=either
  K_omega : Gain  Gain=K_omega*2*pi
  Sum : Sum  Inputs=-+-
  n : Outport
  wires:
  Constant/1 -> Integrator/2
  Integrator/1 -> K_omega/1, n/1
  Finding rotation speed/1 -> Integrator/1
  K_omega/1 -> Sum/3
  Qa/1 -> Sum/1
  Sum/1 -> Finding rotation speed/1
  Qm/1 -> Sum/2

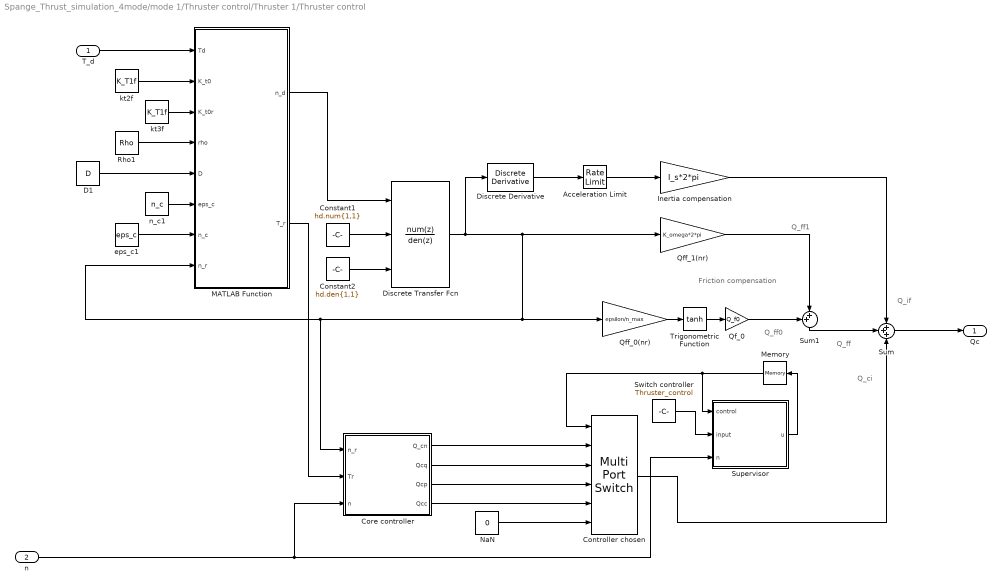
== system Spange_Thrust_simulation_4mode/mode 1/Thruster control/Thruster 1/Thruster control ==
  note: Friction compensation
  note: Q_ff1
  note: Q_ff0
  note: Q_ff
  note: Q_if
  note: Q_ci
  "T_d " : Inport
  n : Inport  Port=2
  Acceleration Limit : RateLimiter  RisingSlewLimit=Max_Acceleration  FallingSlewLimit=-Max_Acceleration  SampleTimeMode=inherited
  Constant1 : Constant  Value=hd.num{1,1}  VectorParams1D=off
  Constant2 : Constant  Value=hd.den{1,1}  VectorParams1D=off
  Controller chosen : MultiPortSwitch  Inputs=5
  Core controller : Subsystem
  D1 : Constant  Value=D  VectorParams1D=off
  Discrete Transfer Fcn : DiscreteTransferFcn  NumeratorSource=Input port  Numerator=[8.76e-05 0.0003481 8.648e-05]  DenominatorSource=Input port  Denominator=[1 -1.974 0.9746]  SampleTime=0.01  a0EqualsOne=on
      settings: InputPortMap=u0,p1,p3
  Discrete Derivative : simulink/Discrete/Discrete Derivative  gainval=1.0  ICPrevScaledInput=0.0  InputProcessing=Inherited  OutMin=[]  OutMax=[]  OutDataType=fixdt(1, 16)  OutScaling=2^-10  DoSatur=off
  Inertia compensation : Gain  Gain=I_s*2*pi
  MATLAB Function : MATLAB Function  TreatAsAtomicUnit=on
  Memory : Memory  X0=1  InheritSampleTime=on
  NaN : Constant  Value=0
  Qf_0 : Gain  Gain=Q_f0
  Qff_0(nr) : Gain  Gain=epsilon/n_max
  Qff_1(nr) : Gain  Gain=K_omega*2*pi
  Rho1 : Constant  Value=Rho  VectorParams1D=off
  Sum : Sum  Inputs=+++
  Sum1 : Sum  Inputs=++|
  Supervisor : MATLAB Function  TreatAsAtomicUnit=on
  Switch controller : Constant  Value=Thruster_control
  Trigonometric Function : Trigonometry  Operator=tanh
  eps_c1 : Constant  Value=eps_c  VectorParams1D=off
  kt2f : Constant  Value=K_T1f  VectorParams1D=off
  kt3f : Constant  Value=K_T1f  VectorParams1D=off
  n_c1 : Constant  Value=n_c  VectorParams1D=off
  Qc : Outport
  wires:
  Sum/1 -> Qc/1
  "T_d "/1 -> MATLAB Function/1(Td)
  Discrete Transfer Fcn/1 -> Discrete Derivative/1, Qff_1(nr)/1, Qff_0(nr)/1, MATLAB Function/8(n_r), Core controller/1(n_r)
  Acceleration Limit/1 -> Inertia compensation/1
  n/1 -> Supervisor/3(n), Core controller/3("n ")
  Inertia compensation/1 -> Sum/1
  Constant2/1 -> Discrete Transfer Fcn/3
  Constant1/1 -> Discrete Transfer Fcn/2
  Sum1/1 -> Sum/2
  Discrete Derivative/1 -> Acceleration Limit/1
  Core controller/1(Q_cn) -> Controller chosen/2
  Core controller/4(Qcc) -> Controller chosen/5
  Core controller/3(Qcp) -> Controller chosen/4
  Core controller/2(Qcq) -> Controller chosen/3
  Controller chosen/1 -> Sum/3
  Switch controller/1 -> Supervisor/2(input)
  Qf_0/1 -> Sum1/1
  Qff_1(nr)/1 -> Sum1/2
  Memory/1 -> Supervisor/1(control), Controller chosen/1
  Supervisor/1(u) -> Memory/1
  NaN/1 -> Controller chosen/6
  Trigonometric Function/1 -> Qf_0/1
  Qff_0(nr)/1 -> Trigonometric Function/1
  MATLAB Function/1(n_d) -> Discrete Transfer Fcn/1
  MATLAB Function/2(T_r) -> Core controller/2("Tr ")
  kt2f/1 -> MATLAB Function/2(K_t0)
  eps_c1/1 -> MATLAB Function/7(n_c)
  D1/1 -> MATLAB Function/5(D)
  Rho1/1 -> MATLAB Function/4(rho)
  kt3f/1 -> MATLAB Function/3(K_t0r)
  n_c1/1 -> MATLAB Function/6(eps_c)

== system Spange_Thrust_simulation_4mode/mode 2/Thruster control/Thruster 1/Propeller Hydrodynamics ==
  env : Inport
  n : Inport  Port=2
  Actual Force and Torque : MATLAB Function  TreatAsAtomicUnit=on
  D1 : Constant  Value=D
  Kq1 : Constant  Value=K_q1f
  Kqr1 : Constant  Value=K_q1r
  Ktf : Constant  Value=K_T1f
  Ktr : Constant  Value=K_T1r
  Rho1 : Constant  Value=Rho
  eps_c1 : Constant  Value=eps_c
  Ta : Outport
  Qa : Outport  Port=2
  wires:
  eps_c1/1 -> Actual Force and Torque/8(eps_c)
  Kqr1/1 -> Actual Force and Torque/5(Kqr)
  Ktr/1 -> Actual Force and Torque/4(Ktr)
  Actual Force and Torque/1(Ta) -> Ta/1
  Ktf/1 -> Actual Force and Torque/3(Kt)
  env/1 -> Actual Force and Torque/9(env)
  Rho1/1 -> Actual Force and Torque/6(Rho)
  Actual Force and Torque/2(Qa) -> Qa/1
  Kq1/1 -> Actual Force and Torque/2(Kq)
  D1/1 -> Actual Force and Torque/7(D)
  n/1 -> Actual Force and Torque/1(n)

== system Spange_Thrust_simulation_4mode/mode 2/Thruster control/Thruster 1/Shaft dynamics ==
  Qm : Inport
  Qa : Inport  Port=2
  Constant : Constant  Value=0
  Finding rotation speed : Gain  Gain=1/(2*pi*I_s)
  Integrator : Integrator  ExternalReset=either
  K_omega : Gain  Gain=K_omega*2*pi
  Sum : Sum  Inputs=-+-
  n : Outport
  wires:
  Constant/1 -> Integrator/2
  Integrator/1 -> K_omega/1, n/1
  Finding rotation speed/1 -> Integrator/1
  K_omega/1 -> Sum/3
  Qa/1 -> Sum/1
  Sum/1 -> Finding rotation speed/1
  Qm/1 -> Sum/2

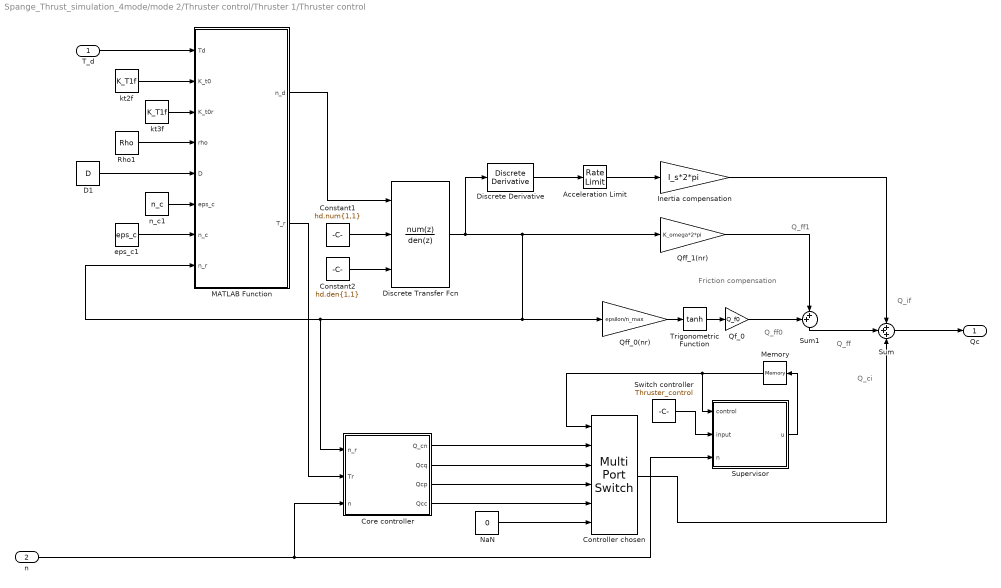
== system Spange_Thrust_simulation_4mode/mode 2/Thruster control/Thruster 1/Thruster control ==
  note: Friction compensation
  note: Q_ff1
  note: Q_ff0
  note: Q_ff
  note: Q_if
  note: Q_ci
  "T_d " : Inport
  n : Inport  Port=2
  Acceleration Limit : RateLimiter  RisingSlewLimit=Max_Acceleration  FallingSlewLimit=-Max_Acceleration  SampleTimeMode=inherited
  Constant1 : Constant  Value=hd.num{1,1}  VectorParams1D=off
  Constant2 : Constant  Value=hd.den{1,1}  VectorParams1D=off
  Controller chosen : MultiPortSwitch  Inputs=5
  Core controller : Subsystem
  D1 : Constant  Value=D  VectorParams1D=off
  Discrete Transfer Fcn : DiscreteTransferFcn  NumeratorSource=Input port  Numerator=[8.76e-05 0.0003481 8.648e-05]  DenominatorSource=Input port  Denominator=[1 -1.974 0.9746]  SampleTime=0.01  a0EqualsOne=on
      settings: InputPortMap=u0,p1,p3
  Discrete Derivative : simulink/Discrete/Discrete Derivative  gainval=1.0  ICPrevScaledInput=0.0  InputProcessing=Inherited  OutMin=[]  OutMax=[]  OutDataType=fixdt(1, 16)  OutScaling=2^-10  DoSatur=off
  Inertia compensation : Gain  Gain=I_s*2*pi
  MATLAB Function : MATLAB Function  TreatAsAtomicUnit=on
  Memory : Memory  X0=1  InheritSampleTime=on
  NaN : Constant  Value=0
  Qf_0 : Gain  Gain=Q_f0
  Qff_0(nr) : Gain  Gain=epsilon/n_max
  Qff_1(nr) : Gain  Gain=K_omega*2*pi
  Rho1 : Constant  Value=Rho  VectorParams1D=off
  Sum : Sum  Inputs=+++
  Sum1 : Sum  Inputs=++|
  Supervisor : MATLAB Function  TreatAsAtomicUnit=on
  Switch controller : Constant  Value=Thruster_control
  Trigonometric Function : Trigonometry  Operator=tanh
  eps_c1 : Constant  Value=eps_c  VectorParams1D=off
  kt2f : Constant  Value=K_T1f  VectorParams1D=off
  kt3f : Constant  Value=K_T1f  VectorParams1D=off
  n_c1 : Constant  Value=n_c  VectorParams1D=off
  Qc : Outport
  wires:
  Sum/1 -> Qc/1
  "T_d "/1 -> MATLAB Function/1(Td)
  Discrete Transfer Fcn/1 -> Discrete Derivative/1, Qff_1(nr)/1, Qff_0(nr)/1, MATLAB Function/8(n_r), Core controller/1(n_r)
  Acceleration Limit/1 -> Inertia compensation/1
  n/1 -> Supervisor/3(n), Core controller/3("n ")
  Inertia compensation/1 -> Sum/1
  Constant2/1 -> Discrete Transfer Fcn/3
  Constant1/1 -> Discrete Transfer Fcn/2
  Sum1/1 -> Sum/2
  Discrete Derivative/1 -> Acceleration Limit/1
  Core controller/1(Q_cn) -> Controller chosen/2
  Core controller/4(Qcc) -> Controller chosen/5
  Core controller/3(Qcp) -> Controller chosen/4
  Core controller/2(Qcq) -> Controller chosen/3
  Controller chosen/1 -> Sum/3
  Switch controller/1 -> Supervisor/2(input)
  Qf_0/1 -> Sum1/1
  Qff_1(nr)/1 -> Sum1/2
  Memory/1 -> Supervisor/1(control), Controller chosen/1
  Supervisor/1(u) -> Memory/1
  NaN/1 -> Controller chosen/6
  Trigonometric Function/1 -> Qf_0/1
  Qff_0(nr)/1 -> Trigonometric Function/1
  MATLAB Function/1(n_d) -> Discrete Transfer Fcn/1
  MATLAB Function/2(T_r) -> Core controller/2("Tr ")
  kt2f/1 -> MATLAB Function/2(K_t0)
  eps_c1/1 -> MATLAB Function/7(n_c)
  D1/1 -> MATLAB Function/5(D)
  Rho1/1 -> MATLAB Function/4(rho)
  kt3f/1 -> MATLAB Function/3(K_t0r)
  n_c1/1 -> MATLAB Function/6(eps_c)

== system Spange_Thrust_simulation_4mode/mode 2/Thruster control/Thruster 3/Propeller Hydrodynamics ==
  env : Inport
  n : Inport  Port=2
  Actual Force and Torque : MATLAB Function  TreatAsAtomicUnit=on
  D : Constant  Value=D
  Kq : Constant  Value=K_q3f
  Kqr : Constant  Value=K_q3r
  Ktf : Constant  Value=K_T3f
  Ktr : Constant  Value=K_T3r
  Rho : Constant  Value=Rho
  eps_c : Constant  Value=eps_c
  Ta : Outport
  Qa : Outport  Port=2
  wires:
  eps_c/1 -> Actual Force and Torque/8(eps_c)
  Kqr/1 -> Actual Force and Torque/5(Kqr)
  Ktr/1 -> Actual Force and Torque/4(Ktr)
  Actual Force and Torque/1(Ta) -> Ta/1
  Ktf/1 -> Actual Force and Torque/3(Kt)
  env/1 -> Actual Force and Torque/9(env)
  Rho/1 -> Actual Force and Torque/6(Rho)
  Actual Force and Torque/2(Qa) -> Qa/1
  Kq/1 -> Actual Force and Torque/2(Kq)
  D/1 -> Actual Force and Torque/7(D)
  n/1 -> Actual Force and Torque/1(n)

== system Spange_Thrust_simulation_4mode/mode 2/Thruster control/Thruster 3/Shaft dynamics ==
  Qm : Inport
  Qa : Inport  Port=2
  Constant : Constant  Value=0
  Finding rotation speed : Gain  Gain=1/(2*pi*I_s)
  Integrator : Integrator  ExternalReset=either
  K_omega : Gain  Gain=K_omega*2*pi
  Sum : Sum  Inputs=-+-
  n : Outport
  wires:
  Constant/1 -> Integrator/2
  Integrator/1 -> K_omega/1, n/1
  Finding rotation speed/1 -> Integrator/1
  K_omega/1 -> Sum/3
  Qa/1 -> Sum/1
  Sum/1 -> Finding rotation speed/1
  Qm/1 -> Sum/2
